simulink model "simmod"  (Simulink 10.1)
settings: Solver=ode45  StartTime=0.0  StopTime=20.0  RelTol=1e-3  EnableMultiTasking=on
values from neighbouring files (symbols this model uses):
  K = param(1)    [PID.m]
  r = double(root(diff(cubicFunc),x))    [KubnaMetoda.m]    (also in PID.m = 0.01)
  Td = param(3)    [PID.m]
  Ti = param(2)    [PID.m]
libraries: cstblocks x1, simulink_need_slupdate x1
settings Model: Creator=Automatika4  LastModifiedBy=Tech
settings DataIOCC: LimitDataPoints=on  SignalLoggingSaveFormat=ModelDataLogs  TimeSaveName=t  OutputSaveName=izlaz
settings OptimizationCC: ExpressionDepthLimit=2147483647
settings DebuggingCC: SolverPrmCheckMsg=warning  FcnCallInpInsideContextMsg=warning  StateNameClashWarn=warning

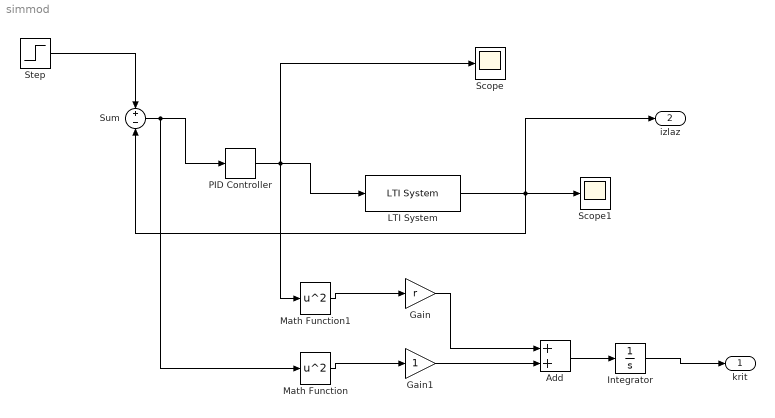
== system simmod ==
  Add : Sum
  Gain : Gain  Gain=r
  Gain1 : Gain
  Integrator : Integrator
  LTI System : cstblocks/LTI System  sys=G  IC=[]
  Math Function : Math  Operator=square  SignedPower=on  SaturateOnIntegerOverflow=on
  Math Function1 : Math  Operator=square  SignedPower=on  SaturateOnIntegerOverflow=on
  PID Controller : simulink_need_slupdate/PID Controller  P=K  I=K/Ti  D=K*Td
  Scope : Scope
  Scope1 : Scope
  Step : Step  Time=0  SampleTime=0
  Sum : Sum  Inputs=+-
  krit : Outport
  izlaz : Outport  Port=2
  wires:
  Add/1 -> Integrator/1
  Integrator/1 -> krit/1
  Gain/1 -> Add/1
  Step/1 -> Sum/1
  LTI System/1 -> Scope1/1, izlaz/1, Sum/2
  Sum/1 -> PID Controller/1, Math Function/1
  PID Controller/1 -> LTI System/1, Math Function1/1, Scope/1
  Math Function1/1 -> Gain/1
  Math Function/1 -> Gain1/1
  Gain1/1 -> Add/2
